simulink model "Model"  (R2018b)
settings: Solver=VariableStepAuto  StartTime=0.0  StopTime=20  FixedStep=0.01  RelTol=1e-3
libraries: robotuavlib x2, robotcorelib x1, aerolibwind2 x1
settings Model: EnablePacing=on  PacingRate=0.110000  Creator=ademuzun  LastModifiedBy=Designer
settings DataIOCC: SaveFormat=Array  ReturnWorkspaceOutputs=on
settings OptimizationCC: SimCompilerOptimization=on
settings HardwareCC: ProdBitPerLong=64  ProdHWDeviceType=Intel->x86-64 (Mac OS X)
settings ModelReferenceCC: EnableParallelModelReferenceBuilds=on  ModelReferenceMinAlgLoopOccurrences=on

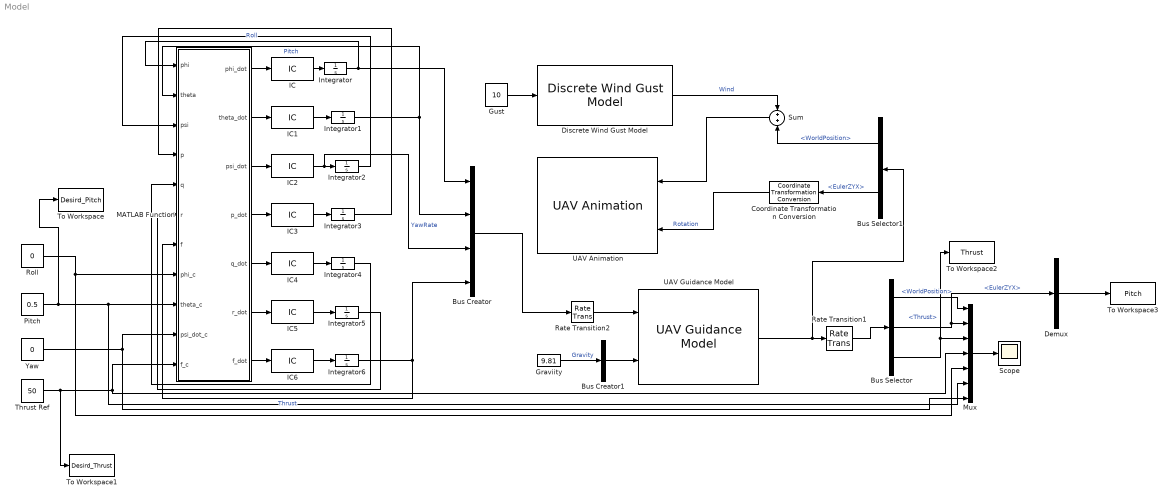
== system Model ==
  Bus Creator : BusCreator  Inputs=4  OutDataTypeStr=Bus: MultirotorGuidanceControlBus  NonVirtualBus=on
  Bus Creator1 : BusCreator  Inputs=1  OutDataTypeStr=Bus: MultirotorGuidanceEnvironmentBus  NonVirtualBus=on
  Bus Selector : BusSelector  OutputSignals=WorldPosition,EulerZYX,Thrust
  Bus Selector1 : BusSelector  OutputSignals=WorldPosition,EulerZYX
  Coordinate Transformation Conversion : robotcorelib/Coordinate Transformation Conversion  InputRepresentation=Euler Angles  InputEulerSequence=ZYX  ShowTrVecInputPort=on  OutputRepresentation=Quaternion  OutputEulerSequence=ZYX  ShowTrVecOutputPort=on  SimulateUsing=Code generation
      settings: SourceProductBaseCode=RO
  Demux : Demux  Outputs=3
  Discrete Wind Gust Model : aerolibwind2/Discrete Wind Gust Model  units=Metric (MKS)  Gx=on  Gy=on  Gz=on  t_0=0.1  d_m=[120 120 80]  v_m=[3.5 3.5 3.0]
      settings: SourceProductName=Aerospace Blockset
  Graviity : Constant  Value=9.81
  Gust : Constant  Value=10
  IC{,1..6} (7 alike) : InitialCondition  Value=0.00001
  Integrator{,1..6} (7 alike) : Integrator
  MATLAB Function : MATLAB Function  TreatAsAtomicUnit=on
  Mux : Mux  Inputs=7
  Pitch : Constant  Value=0.5
  Rate Transition1 : RateTransition  OutPortSampleTime=0.01
  Rate Transition2 : RateTransition  OutPortSampleTime=0.1
  Roll : Constant  Value=0
  Scope : Scope
  Sum : Sum  Inputs=+|+
  Thrust Ref : Constant  Value=50
  To Workspace : ToWorkspace  VariableName=Desird_Pitch  SaveFormat=Timeseries  SampleTime=-1
  To Workspace1 : ToWorkspace  VariableName=Desird_Thrust  SaveFormat=Timeseries  SampleTime=-1
  To Workspace2 : ToWorkspace  VariableName=Thrust  SaveFormat=Timeseries  SampleTime=-1
  To Workspace3 : ToWorkspace  VariableName=Pitch  SaveFormat=Timeseries  SampleTime=-1
  UAV Animation : robotuavlib/UAV Animation  UAVType=Multirotor  UAVSize=1  InertialZDirection=Down  SampleTime=-1
      settings: SourceProductName=Robotics System Toolbox UAV Library  SourceProductBaseCode=ROBOTICS_UAV_LIB
  UAV Guidance Model : robotuavlib/UAV Guidance Model  ModelType=MultirotorGuidance  SpecifiedDataType=double  SimulateUsing=Interpreted execution  InitialWorldPositionMultirotor=[0; 0; 0]  InitialWorldVelocityMultirotor=[0; 0; 0]  InitialEulerZYXMultirotor=[0; 0; 0]  InitialBodyAngularRateRPYMultirotor=[0; 0; 0]  InitialThrustMultirotor=0  InitialNorthFixedWing=0  InitialEastFixedWing=0  InitialHeightFixedWing=0  InitialAirSpeedFixedWing=0  InitialHeadingAngleFixedWing=0  InitialFlightPathAngleFixedWing=0  InitialRollAngleFixedWing=0  InitialRollAngleRateFixedWing=0  PDRollMultirotor=[3402.97,116.67]  PDPitchMultirotor=[3402.97, 116.67]  PYawRateMultirotor=1950  PThrustMultirotor=3900  MassMultirotor=0.5  PHeightFixedWing=3.9  PHeadingAngleFixedWing=3.9  PFlightPathAngleFixedWing=39  PDRollFixedWing=[3402.97, 116.67]  PAirSpeedFixedWing=1  FlightPathAngleLimitsFixedWing=[-pi/2, pi/2]  StateBusName='MultirotorGuidanceStateBus'  ControlBusName='MultirotorGuidanceControlBus'  EnvironmentBusName='MultirotorGuidanceEnvironmentBus'  DataType=double
      settings: SourceProductName=Robotics System Toolbox UAV Library  SourceProductBaseCode=ROBOTICS_UAV_LIB
  Yaw : Constant  Value=0
  wires:
  Bus Selector/1 -> Mux/1  "<WorldPosition>"
  Rate Transition2/1 -> UAV Guidance Model/1
  Bus Creator/1 -> Rate Transition2/1
  Graviity/1 -> Bus Creator1/1  "Gravity"
  UAV Guidance Model/1 -> Rate Transition1/1, Bus Selector1/1
  Rate Transition1/1 -> Bus Selector/1
  Bus Selector/2 -> Demux/1, Mux/2  "<EulerZYX>"
  Bus Creator1/1 -> UAV Guidance Model/2
  Bus Selector1/2 -> Coordinate Transformation Conversion/1  "<EulerZYX>"
  Coordinate Transformation Conversion/1 -> UAV Animation/2  "Rotation"
  Bus Selector/3 -> To Workspace2/1, Mux/3  "<Thrust>"
  Integrator/1 -> MATLAB Function/1(phi), Bus Creator/1  "Roll"
  Integrator1/1 -> MATLAB Function/2(theta), Bus Creator/2  "Pitch"
  IC2/1 -> Bus Creator/3, Integrator2/1  "YawRate"
  Integrator6/1 -> Bus Creator/4, MATLAB Function/7(f)  "Thrust"
  MATLAB Function/1(phi_dot) -> IC/1
  IC6/1 -> Integrator6/1
  IC4/1 -> Integrator4/1
  Integrator2/1 -> MATLAB Function/3(psi)
  MATLAB Function/6(r_dot) -> IC5/1
  MATLAB Function/7(f_dot) -> IC6/1
  Integrator3/1 -> MATLAB Function/4(p)
  MATLAB Function/2(theta_dot) -> IC1/1
  Integrator4/1 -> MATLAB Function/5(q)
  MATLAB Function/4(p_dot) -> IC3/1
  MATLAB Function/5(q_dot) -> IC4/1
  IC/1 -> Integrator/1
  IC5/1 -> Integrator5/1
  Integrator5/1 -> MATLAB Function/6(r)
  MATLAB Function/3(psi_dot) -> IC2/1
  IC1/1 -> Integrator1/1
  IC3/1 -> Integrator3/1
  Yaw/1 -> MATLAB Function/10(psi_dot_c), Mux/7
  Thrust Ref/1 -> To Workspace1/1, MATLAB Function/11(f_c), Mux/4
  Mux/1 -> Scope/1
  Pitch/1 -> To Workspace/1, Mux/6, MATLAB Function/9(theta_c)
  Roll/1 -> Mux/5, MATLAB Function/8(phi_c)
  Sum/1 -> UAV Animation/1
  Gust/1 -> Discrete Wind Gust Model/1
  Bus Selector1/1 -> Sum/2  "<WorldPosition>"
  Discrete Wind Gust Model/1 -> Sum/1  "Wind"
  Demux/2 -> To Workspace3/1

== matlab function Model/MATLAB Function ==
  data: phi input; phi_dot output; theta_dot output; psi_dot output; p_dot output; q_dot output; r_dot output; theta input; psi input; p input; q input; r input; f input; phi_c input; theta_c input; psi_dot_c input; f_dot output; f_c input
function [phi_dot,theta_dot,psi_dot,p_dot,q_dot,r_dot,f_dot]= UAV_model(phi,theta,psi,p,q,r,f,phi_c,theta_c,psi_dot_c,f_c)
% Tuned Kp and Kd constants for PD controller
Kp_phi= 3400; Kp_theta= 3400; Kp_psi= 1900; Kp_f=3900; Kd_phi=115; Kd_theta=115;
% Implementation for system states
x1= phi;
x3= theta;
x5= psi;
x7= p;
x9= q;
x11= r;
x13=f;
x2=x7+sin(x1)*tan(x3)*x9+cos(x1)*tan(x3)*x11;
x4=cos(x1)*x9-sin(x1)*x11;
x6=sin(x1)/cos(x3)*x9+cos(x1)/cos(x3)*x11;
x8=Kp_phi*(phi_c-x1)+Kd_phi*(-x2)-sin(x3)*Kp_psi*(psi_dot_c-x6);
x10=cos(x1)*(Kp_theta*(theta_c-x3)+Kd_theta*(-x4))+sin(x1)*cos(x3)*Kp_psi*(psi_dot_c-x6);
x12=-sin(x1)*(Kp_theta*(theta_c-x3)+Kd_theta*(-x4))+cos(x1)*cos(x3)*Kp_psi*(psi_dot_c-x6);
x14=Kp_f*(f_c-x13);

% outputs
phi_dot=x2;
theta_dot=x4;
psi_dot=x6;
p_dot=x8;
q_dot=x10;
r_dot=x12;
f_dot=x14;

end
